simulink library "INT_PIntkVUs_DD"  (R2016b)
settings: Solver=VariableStepAuto  StartTime=0.0  StopTime=10.0  RelTol=1e-3
settings Model: Creator=Administrator  LastModifiedBy=Administrator

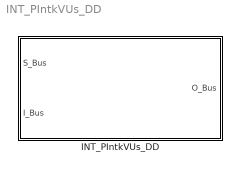
== system INT_PIntkVUs_DD ==
  INT_PIntkVUs_DD : Subsystem

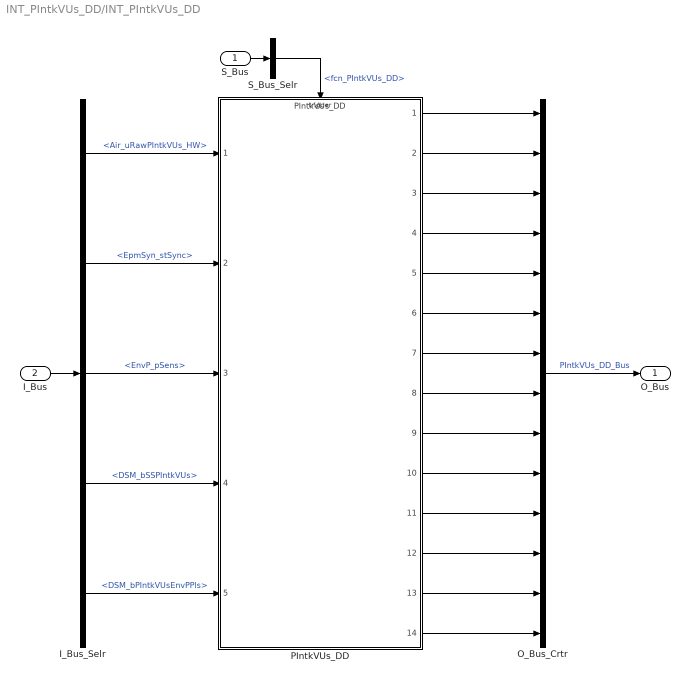
== system INT_PIntkVUs_DD/INT_PIntkVUs_DD ==
  S_Bus : Inport
  I_Bus : Inport  Port=2
  I_Bus_Selr : BusSelector  OutputSignals=Air_uRawPIntkVUs_HW,EpmSyn_stSync,EnvP_pSens,DSM_bSSPIntkVUs,DSM_bPIntkVUsEnvPPls
  O_Bus_Crtr : BusCreator  Inputs=14
  PIntkVUs_DD : ModelReference  ModelNameDialog=PIntkVUs_DD  SimulationMode=Normal  ModelReferenceVersion=1.44  TriggerPortName=function  TriggerPortTriggerType=function-call  TriggerPortStatesWhenEnabling=held
  S_Bus_Selr : BusSelector  OutputSignals=fcn_PIntkVUs_DD
  O_Bus : Outport
  wires:
  S_Bus_Selr/1 -> PIntkVUs_DD/Trigger  "<fcn_PIntkVUs_DD>"
  S_Bus/1 -> S_Bus_Selr/1
  I_Bus/1 -> I_Bus_Selr/1
  I_Bus_Selr/1 -> PIntkVUs_DD/1  "<Air_uRawPIntkVUs_HW>"
  I_Bus_Selr/2 -> PIntkVUs_DD/2  "<EpmSyn_stSync>"
  I_Bus_Selr/3 -> PIntkVUs_DD/3  "<EnvP_pSens>"
  I_Bus_Selr/4 -> PIntkVUs_DD/4  "<DSM_bSSPIntkVUs>"
  I_Bus_Selr/5 -> PIntkVUs_DD/5  "<DSM_bPIntkVUsEnvPPls>"
  O_Bus_Crtr/1 -> O_Bus/1  "PIntkVUs_DD_Bus"
  PIntkVUs_DD/1 -> O_Bus_Crtr/1
  PIntkVUs_DD/2 -> O_Bus_Crtr/2
  PIntkVUs_DD/3 -> O_Bus_Crtr/3
  PIntkVUs_DD/4 -> O_Bus_Crtr/4
  PIntkVUs_DD/5 -> O_Bus_Crtr/5
  PIntkVUs_DD/6 -> O_Bus_Crtr/6
  PIntkVUs_DD/7 -> O_Bus_Crtr/7
  PIntkVUs_DD/8 -> O_Bus_Crtr/8
  PIntkVUs_DD/9 -> O_Bus_Crtr/9
  PIntkVUs_DD/10 -> O_Bus_Crtr/10
  PIntkVUs_DD/11 -> O_Bus_Crtr/11
  PIntkVUs_DD/12 -> O_Bus_Crtr/12
  PIntkVUs_DD/13 -> O_Bus_Crtr/13
  PIntkVUs_DD/14 -> O_Bus_Crtr/14
